simulink model "AttitudeController"  (R2018b)
settings: Solver=VariableStepAuto  StartTime=0.0  StopTime=15000  FixedStep=1  RelTol=1e-2
values from neighbouring files (symbols this model uses):
  torquemax = cross(grate,If*wf')    [controller.m]
  wCyc = [0,0,sqrt(g/l)]    [MomentOfInertia.m]
  ZTorqueBev = 1.0564    [CMGsizing.m]
undefined symbols (not defined in the file or in its folder): ICycler3
libraries: simulink x1
settings Model: Creator=rfrankl  LastModifiedBy=rfrankl
settings SolverCC: AlgebraicLoopSolver=LineSearch
settings DebuggingCC: AlgebraicLoopMsg=none

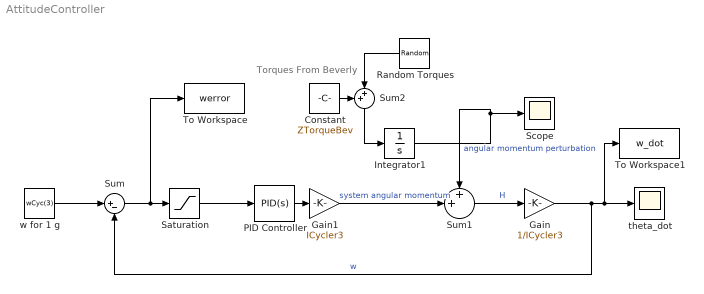
== system AttitudeController ==
  note: Torques From Beverly
  Constant : Constant  Value=ZTorqueBev
  Gain : Gain  Gain=1/ICycler3
  Gain1 : Gain  Gain=ICycler3
  Integrator1 : Integrator
  PID Controller : simulink/Continuous/PID Controller  Controller=PID  Form=Parallel  TimeDomain=Continuous-time  SampleTime=-1  IntegratorMethod=Forward Euler  FilterMethod=Forward Euler  ControllerParametersSource=internal  P=0  I=100  D=0  UseFilter=on  N=100  TunerSelectOption=Transfer Function Based (PID Tuner App)  InitialConditionSource=internal  InitialConditionForIntegrator=0  InitialConditionForFilter=0  DifferentiatorICPrevScaledInput=0  ExternalReset=none  TrackingMode=off  Kt=1  LimitOutput=off  UpperSaturationLimit=inf  LowerSaturationLimit=-inf  LinearizeAsGain=on  AntiWindupMode=none  Kb=1  POutMin=[]  POutMax=[]  IOutMin=[]  IOutMax=[]  DOutMin=[]  DOutMax=[]  NOutMin=[]  NOutMax=[]  SumOutMin=[]  SumOutMax=[]  SaturationOutMin=[]  SaturationOutMax=[]  PParamMin=[]  PParamMax=[]  IParamMin=[]  IParamMax=[]  DParamMin=[]  DParamMax=[]  NParamMin=[]  NParamMax=[]  KbParamMin=[]  KbParamMax=[]  KtParamMin=[]  KtParamMax=[]  KbOutMin=[]  KbOutMax=[]  KtOutMin=[]  KtOutMax=[]  IntegratorOutMin=[]  IntegratorOutMax=[]  FilterOutMin=[]  FilterOutMax=[]  SumI1OutMin=[]  SumI1OutMax=[]  SumI2OutMin=[]  SumI2OutMax=[]  SumI3OutMin=[]  SumI3OutMax=[]  SumI4OutMin=[]  SumI4OutMax=[]  SumDOutMin=[]  SumDOutMax=[]  DifferentiatorOutMin=[]  DifferentiatorOutMax=[]  FilterDiffOutCoefMin=[]  FilterDiffOutCoefMax=[]  ReciprocalOutMin=[]  ReciprocalOutMax=[]  SumDenOutMin=[]  SumDenOutMax=[]  SumNumOutMin=[]  SumNumOutMax=[]  DivideOutMin=[]  DivideOutMax=[]  IntegratorContinuousStateAttributes=''  IntegratorStateMustResolveToSignalObject=off  IntegratorRTWStateStorageClass=Auto  FilterContinuousStateAttributes=''  FilterStateMustResolveToSignalObject=off  FilterRTWStateStorageClass=Auto  ParallelPVariant=InternalParameters  IdealPVariant=Disabled  IVariant=InternalParameters  DVariant=InternalParameters  IntegratorVariant=Continuous  SatVariant=Disabled  AWVariant=Passthrough  PCopyVariant=Disabled  TRVariant=Disabled  FdbkBlocksVariant=Forward  IdealPFdbkVariant=Disabled  SatFdbkVariant=Disabled  DerivativeFilterVariant=ContFilter  NVariant=InternalParameters  NCopyVariant=Disabled  FilterICVariant=InternalICsFilter  IntegratorICVariant=InternalICs  ExternalResetVariant=Disabled  TRSumVariant=Passthrough  SumFdbkVariant=Disabled  SumVariant=Sum_PID
  Random Torques : RandomNumber  Mean=10  SampleTime=1
  Saturation : Saturate  UpperLimit=torquemax(1) * .15/ICycler3  LowerLimit=-torquemax(1) * .15/ICycler3
  Scope : Scope
  Sum : Sum  Inputs=|+-
  Sum1 : Sum  Inputs=++|
  Sum2 : Sum  Inputs=++|
  To Workspace : ToWorkspace  VariableName=werror  SaveFormat=Timeseries  SampleTime=-1
  To Workspace1 : ToWorkspace  VariableName=w_dot  SaveFormat=Timeseries  SampleTime=-1
  theta_dot : Scope
  w for 1 g : Constant  Value=wCyc(3)
  wires:
  Gain/1 -> theta_dot/1, To Workspace1/1, Sum/2  "w"
  w for 1 g/1 -> Sum/1
  Sum1/1 -> Gain/1  "H"
  Gain1/1 -> Sum1/2  "system angular momentum"
  Sum2/1 -> Integrator1/1
  Constant/1 -> Sum2/1
  Integrator1/1 -> Sum1/1, Scope/1  "angular momentum perturbation"
  PID Controller/1 -> Gain1/1
  Sum/1 -> To Workspace/1, Saturation/1
  Saturation/1 -> PID Controller/1
  Random Torques/1 -> Sum2/2
